simulink model "Asg3_2_linear"  (R2020b)
settings: Solver=VariableStepAuto  StartTime=0.0  StopTime=10.0  RelTol=1e-3
settings Model: Creator=Master  LastModifiedBy=Pratyush Jaiswal
settings DebuggingCC: SFMachineParentedDataDiag=error

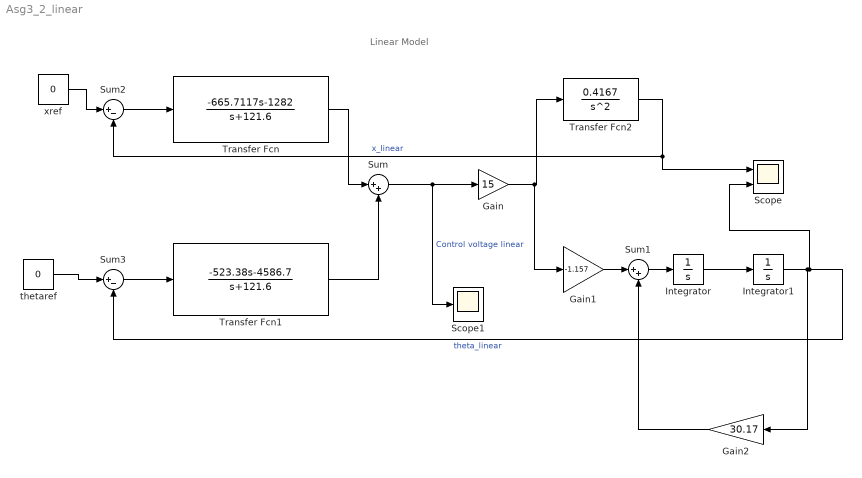
== system Asg3_2_linear ==
  note: Linear Model
  Gain : Gain  Gain=15
  Gain1 : Gain  Gain=-1.157
  Gain2 : Gain  Gain=30.17
  Integrator : Integrator
  Integrator1 : Integrator  InitialCondition=0.15
  Scope : Scope  NumInputPorts=2
  Scope1 : Scope
  Sum : Sum  Inputs=|++
  Sum1 : Sum  Inputs=|++
  Sum2 : Sum  Inputs=|+-
  Sum3 : Sum  Inputs=|+-
  Transfer Fcn : TransferFcn  Numerator=[-665.7117 -1282]  Denominator=[1 121.6]
  Transfer Fcn1 : TransferFcn  Numerator=[-523.38 -4586.7]  Denominator=[1 121.6]
  Transfer Fcn2 : TransferFcn  Numerator=[0.4167]  Denominator=[1 0 0]
  thetaref : Constant  Value=0
  xref : Constant  Value=0
  wires:
  Sum3/1 -> Transfer Fcn1/1
  xref/1 -> Sum2/1
  Sum/1 -> Scope1/1, Gain/1  "Control voltage linear"
  Gain1/1 -> Sum1/1
  thetaref/1 -> Sum3/1
  Sum2/1 -> Transfer Fcn/1
  Integrator1/1 -> Scope/2, Sum3/2, Gain2/1  "theta_linear"
  Gain/1 -> Gain1/1, Transfer Fcn2/1
  Sum1/1 -> Integrator/1
  Integrator/1 -> Integrator1/1
  Transfer Fcn2/1 -> Sum2/2, Scope/1  "x_linear"
  Gain2/1 -> Sum1/2
  Transfer Fcn1/1 -> Sum/2
  Transfer Fcn/1 -> Sum/1
